simulink model "LATC_Test_Calc"  (R2021b)
settings: Solver=FixedStepDiscrete  StartTime=0.0  StopTime=inf  FixedStep=0.01  RelTol=1e-3
undefined symbols (not defined in the file or in its folder): P_LCS_A0_Dis_BP, P_LCS_A2_Curve_BP, P_LCS_A2S_FliterTime, P_LCS_DeltaEps_SpdBp, P_LCS_LCC_A0_Dis_BP, P_LCS_LCC_AngleSlope_ELK, P_LCS_LCC_AngleSlope_ESS, P_LCS_LCC_AngleSlope_LCCancle, P_LCS_LCC_AngleSlope_LCEco, P_LCS_LCC_AngleSlope_LCK, P_LCS_LCC_AngleSlope_LCKIE, P_LCS_LCC_AngleSlope_LCNomal, P_LCS_LCC_AngleSlope_LCSport, P_LCS_LCC_AngleSlope_LKA, P_LCS_LCC_Eco_AyDtLimit_TBL, P_LCS_LCC_ELK_AyDtLimit_TBL, P_LCS_LCC_ESS_AyDtLimit_TBL, P_LCS_LCC_LC_AyDtLimit_TBL, P_LCS_LCC_LC_Normal_AyDtLimit_TBL, P_LCS_LCC_LC_Planning_Dist_TBL, P_LCS_LCC_LCK_AyDtLimit_TBL, P_LCS_LCC_LCK_Planning_Dist_TBL, P_LCS_LCC_LKA_AyDtLimit_TBL, P_LCS_LCC_Matrix_q1_st, P_LCS_LCC_Matrix_q2_st, P_LCS_LCC_Max_Lateral_Acc_ms2, P_LCS_LCC_MaxLatAcc_ELK, P_LCS_LCC_MaxLatAcc_ESS, P_LCS_LCC_MaxLatAcc_LCCancel, P_LCS_LCC_MaxLatAcc_LCEco, P_LCS_LCC_MaxLatAcc_LCK, P_LCS_LCC_MaxLatAcc_LCKIE, P_LCS_LCC_MaxLatAcc_LCNomal, P_LCS_LCC_MaxLatAcc_LCSport, P_LCS_LCC_MaxLatAcc_LKA, P_LCS_LCC_Min_Plan_Dis, P_LCS_LCC_PlaningLength_m, P_LCS_LCC_PreCur_Min_Plan_Dis_Fac, P_LCS_LCC_PreView_Fac, P_LCS_LCC_PreView_s, P_LCS_LCC_PreViewCurve_Fac, P_LCS_LCC_PreViewT, P_LCS_LCC_Spd_BP, P_LCS_LCC_Spd_BP2, P_LCS_LCC_Sport_AyDtLimit_TBL, P_LCS_LCC_StateActiv_AyDtLimit, P_LCS_LCC_StateActiv_PreviewT, P_LCS_LCC_StateActiveDelaytime, P_LCS_LCC_TarSteerAngleSlope, P_LCS_preDis_spd, P_LCS_StateActiv_AngleSlope, P_LCS_StateActive_HoldTime_BP, P_LCS_StateActiveFlg_BP, P_LCS_StateHold_time
libraries: canapelib x35, simulink x2
(part 2 of 3)

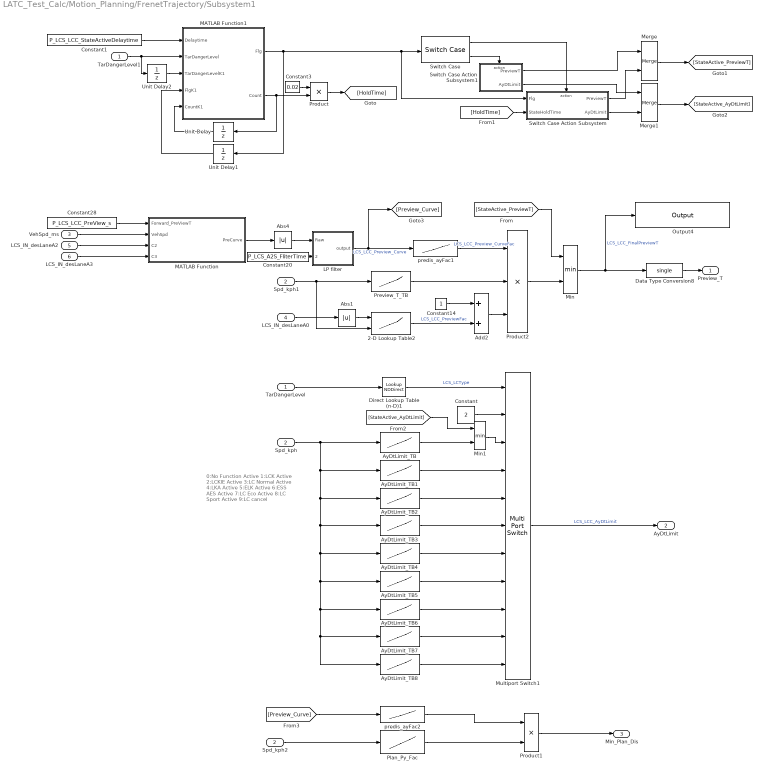
== system LATC_Test_Calc/Motion_Planning/FrenetTrajectory/Subsystem1 ==
  note: 0:No Function Active
      | 1:LCK Active
      | 2:LCKIE Active
      | 3:LC Normal Active
      | 4:LKA Active
      | 5:ELK Active
      | 6:ESS AES Active
      | 7:LC Eco Active
      | 8:LC Sport Active
      | 9:LC cancel
  TarDangerLevel : Inport
  Spd_kph : Inport  Port=2
  VehSpd_ms : Inport  Port=3
  LCS_IN_desLaneA0 : Inport  Port=4
  LCS_IN_desLaneA2 : Inport  Port=5
  LCS_IN_desLaneA3 : Inport  Port=6
  2-D Lookup Table2 : Lookup_n-D  BreakpointsForDimension1=P_LCS_A0_Dis_BP  BreakpointsForDimension2=P_LCS_preDis_spd  Table=P_LCS_LCC_PreView_Fac  ExtrapMethod=Clip  UseLastTableValue=on  InternalRulePriority=Speed  RndMeth=Simplest  InputSameDT=on
      settings: InputPortMap=u0,u1
  Abs1 : Abs
  Abs4 : Abs
  Add2 : Sum
  AyDtLimit_TB : Lookup_n-D  NumberOfTableDimensions=1  BreakpointsForDimension1=P_LCS_preDis_spd  Table=P_LCS_LCC_LCK_AyDtLimit_TBL  ExtrapMethod=Clip  UseLastTableValue=on  InternalRulePriority=Speed  RndMeth=Simplest  InputSameDT=on
  AyDtLimit_TB1 : Lookup_n-D  NumberOfTableDimensions=1  BreakpointsForDimension1=P_LCS_preDis_spd  Table=P_LCS_LCC_LCK_AyDtLimit_TBL  ExtrapMethod=Clip  UseLastTableValue=on  InternalRulePriority=Speed  RndMeth=Simplest  InputSameDT=on
  AyDtLimit_TB2 : Lookup_n-D  NumberOfTableDimensions=1  BreakpointsForDimension1=P_LCS_preDis_spd  Table=P_LCS_LCC_LC_Normal_AyDtLimit_TBL  ExtrapMethod=Clip  UseLastTableValue=on  InternalRulePriority=Speed  RndMeth=Simplest  InputSameDT=on
  AyDtLimit_TB3 : Lookup_n-D  NumberOfTableDimensions=1  BreakpointsForDimension1=P_LCS_preDis_spd  Table=P_LCS_LCC_LKA_AyDtLimit_TBL  ExtrapMethod=Clip  UseLastTableValue=on  InternalRulePriority=Speed  RndMeth=Simplest  InputSameDT=on
  AyDtLimit_TB4 : Lookup_n-D  NumberOfTableDimensions=1  BreakpointsForDimension1=P_LCS_preDis_spd  Table=P_LCS_LCC_ELK_AyDtLimit_TBL  ExtrapMethod=Clip  UseLastTableValue=on  InternalRulePriority=Speed  RndMeth=Simplest  InputSameDT=on
  AyDtLimit_TB5 : Lookup_n-D  NumberOfTableDimensions=1  BreakpointsForDimension1=P_LCS_preDis_spd  Table=P_LCS_LCC_ESS_AyDtLimit_TBL  ExtrapMethod=Clip  UseLastTableValue=on  InternalRulePriority=Speed  RndMeth=Simplest  InputSameDT=on
  AyDtLimit_TB6 : Lookup_n-D  NumberOfTableDimensions=1  BreakpointsForDimension1=P_LCS_preDis_spd  Table=P_LCS_LCC_Eco_AyDtLimit_TBL  ExtrapMethod=Clip  UseLastTableValue=on  InternalRulePriority=Speed  RndMeth=Simplest  InputSameDT=on
  AyDtLimit_TB7 : Lookup_n-D  NumberOfTableDimensions=1  BreakpointsForDimension1=P_LCS_preDis_spd  Table=P_LCS_LCC_Sport_AyDtLimit_TBL  ExtrapMethod=Clip  UseLastTableValue=on  InternalRulePriority=Speed  RndMeth=Simplest  InputSameDT=on
  AyDtLimit_TB8 : Lookup_n-D  NumberOfTableDimensions=1  BreakpointsForDimension1=P_LCS_preDis_spd  Table=P_LCS_LCC_LC_AyDtLimit_TBL  ExtrapMethod=Clip  UseLastTableValue=on  InternalRulePriority=Speed  RndMeth=Simplest  InputSameDT=on
  Constant : Constant  Value=2  OutDataTypeStr=single
  Constant1 : Constant  Value=P_LCS_LCC_StateActiveDelaytime  OutDataTypeStr=uint16
  Constant14 : Constant  OutDataTypeStr=single
  Constant20 : Constant  Value=P_LCS_A2S_FliterTime
  Constant28 : Constant  Value=P_LCS_LCC_PreView_s  OutDataTypeStr=single
  Constant3 : Constant  Value=0.02
  Data Type Conversion8 : DataTypeConversion  OutDataTypeStr=single
  Direct Lookup Table (n-D)1 : LookupNDDirect  NumberOfTableDimensions=1  Table=[0 1 2 3 4 5 6 7 8 9]  TableDataTypeStr=uint8
  LP filter : Subsystem
  MATLAB Function : MATLAB Function  TreatAsAtomicUnit=on
  MATLAB Function1 : MATLAB Function  TreatAsAtomicUnit=on
  Merge : Merge
  Merge1 : Merge
  Min : MinMax  Inputs=2
  Min1 : MinMax  Inputs=2
  Multiport Switch1 : MultiPortSwitch  DataPortOrder=Zero-based contiguous  Inputs=10  zeroidx=on
  Output4 : canapelib/CANape I//O/Output  envName=LCS_LCC_FinalPreviewT  envRows=1  envCols=1  envPortId=0
      settings: AttributesFormatString=%<envName>  SourceProductName=Vector CANape/vSignalyzer Target
  Plan_Py_Fac : Lookup_n-D  NumberOfTableDimensions=1  BreakpointsForDimension1=P_LCS_DeltaEps_SpdBp  Table=P_LCS_LCC_Min_Plan_Dis  ExtrapMethod=Clip  UseLastTableValue=on  InternalRulePriority=Speed  RndMeth=Simplest  InputSameDT=on
  Preview_T_TB : Lookup_n-D  NumberOfTableDimensions=1  BreakpointsForDimension1=P_LCS_preDis_spd  Table=P_LCS_LCC_PreViewT  ExtrapMethod=Clip  UseLastTableValue=on  InternalRulePriority=Speed  RndMeth=Simplest  InputSameDT=on
  Product : Product
  Product1 : Product
  Product2 : Product  Inputs=3
  Spd_kph1 : InportShadow  Port=2
  Spd_kph2 : InportShadow  Port=2
  Switch Case : SwitchCase  CaseConditions={[1]}
  Switch Case Action Subsystem : Subsystem  TreatAsAtomicUnit=on
  Switch Case Action Subsystem1 : Subsystem  TreatAsAtomicUnit=on
  TarDangerLevel1 : InportShadow
  Unit Delay : UnitDelay  SampleTime=-1  HasFrameUpgradeWarning=on
  Unit Delay1 : UnitDelay  SampleTime=-1  HasFrameUpgradeWarning=on
  Unit Delay2 : UnitDelay  SampleTime=-1  HasFrameUpgradeWarning=on
  predis_ayFac1 : Lookup_n-D  NumberOfTableDimensions=1  BreakpointsForDimension1=P_LCS_A2_Curve_BP  Table=P_LCS_LCC_PreViewCurve_Fac  ExtrapMethod=Clip  UseLastTableValue=on  InternalRulePriority=Speed  RndMeth=Simplest  InputSameDT=on
  predis_ayFac2 : Lookup_n-D  NumberOfTableDimensions=1  BreakpointsForDimension1=P_LCS_A2_Curve_BP  Table=P_LCS_LCC_PreCur_Min_Plan_Dis_Fac  ExtrapMethod=Clip  UseLastTableValue=on  InternalRulePriority=Speed  RndMeth=Simplest  InputSameDT=on
  Preview_T : Outport  OutDataTypeStr=single
  AyDtLimit : Outport  Port=2  OutDataTypeStr=single
  Min_Plan_Dis : Outport  Port=3  OutDataTypeStr=single
  wires:
  Min1/1 -> Multiport Switch1/3
  [StateActive_AyDtLimit] -> Min1/1
  Product2/1 -> Min/2
  [StateActive_PreviewT] -> Min/1
  Merge1/1 -> [StateActive_AyDtLimit]
  Merge/1 -> [StateActive_PreviewT]
  Switch Case Action Subsystem1/2(AyDtLimit) -> Merge1/1
  Switch Case Action Subsystem/2(AyDtLimit) -> Merge1/2
  Product/1 -> [HoldTime]
  [HoldTime] -> Switch Case Action Subsystem/2(StateHoldTime)
  Constant3/1 -> Product/1
  Switch Case/2 -> Switch Case Action Subsystem1/Action
  MATLAB Function1/2(Count) -> Unit Delay/1, Product/2
  Switch Case Action Subsystem/1(PreviewT) -> Merge/2
  Switch Case/1 -> Switch Case Action Subsystem/Action
  Switch Case Action Subsystem1/1(PreviewT) -> Merge/1
  MATLAB Function1/1(Flg) -> Switch Case/1, Switch Case Action Subsystem/1(Flg), Unit Delay1/1
  Constant1/1 -> MATLAB Function1/1(Delaytime)
  Unit Delay2/1 -> MATLAB Function1/3(TarDangerLevelK1)
  TarDangerLevel1/1 -> MATLAB Function1/2(TarDangerLevel), Unit Delay2/1
  Unit Delay1/1 -> MATLAB Function1/4(FlgK1)
  Unit Delay/1 -> MATLAB Function1/5(CountK1)
  AyDtLimit_TB8/1 -> Multiport Switch1/11
  AyDtLimit_TB7/1 -> Multiport Switch1/10
  AyDtLimit_TB6/1 -> Multiport Switch1/9
  AyDtLimit_TB5/1 -> Multiport Switch1/8
  AyDtLimit_TB4/1 -> Multiport Switch1/7
  AyDtLimit_TB3/1 -> Multiport Switch1/6
  AyDtLimit_TB2/1 -> Multiport Switch1/5
  AyDtLimit_TB1/1 -> Multiport Switch1/4
  Constant/1 -> Multiport Switch1/2
  Constant28/1 -> MATLAB Function/1(Forward_PreViewT)
  predis_ayFac1/1 -> Product2/1  "LCS_LCC_Preview_CurveFac"
  LP filter/1(output) -> [Preview_Curve], predis_ayFac1/1  "LCS_LCC_Preview_Curve"
  Constant20/1 -> LP filter/2(TorqFilterTime)
  Abs4/1 -> LP filter/1(Raw)
  MATLAB Function/1(PreCurve) -> Abs4/1
  LCS_IN_desLaneA3/1 -> MATLAB Function/4(C3)
  LCS_IN_desLaneA2/1 -> MATLAB Function/3(C2)
  VehSpd_ms/1 -> MATLAB Function/2(VehSpd)
  Data Type Conversion8/1 -> Preview_T/1
  Min/1 -> Output4/1, Data Type Conversion8/1  "LCS_LCC_FinalPreviewT"
  LCS_IN_desLaneA0/1 -> Abs1/1
  Abs1/1 -> 2-D Lookup Table2/1
  Spd_kph1/1 -> Preview_T_TB/1, 2-D Lookup Table2/2
  Add2/1 -> Product2/3
  Constant14/1 -> Add2/1
  2-D Lookup Table2/1 -> Add2/2  "LCS_LCC_PreviewFac"
  Preview_T_TB/1 -> Product2/2
  AyDtLimit_TB/1 -> Min1/2
  Multiport Switch1/1 -> AyDtLimit/1  "LCS_LCC_AyDtLimit"
  Spd_kph/1 -> AyDtLimit_TB/1, AyDtLimit_TB1/1, AyDtLimit_TB2/1, AyDtLimit_TB4/1, AyDtLimit_TB5/1, AyDtLimit_TB7/1, AyDtLimit_TB8/1, AyDtLimit_TB6/1, AyDtLimit_TB3/1
  TarDangerLevel/1 -> Direct Lookup Table (n-D)1/1
  Direct Lookup Table (n-D)1/1 -> Multiport Switch1/1  "LCS_LCType"
  Plan_Py_Fac/1 -> Product1/2
  Spd_kph2/1 -> Plan_Py_Fac/1
  [Preview_Curve] -> predis_ayFac2/1
  Product1/1 -> Min_Plan_Dis/1
  predis_ayFac2/1 -> Product1/1

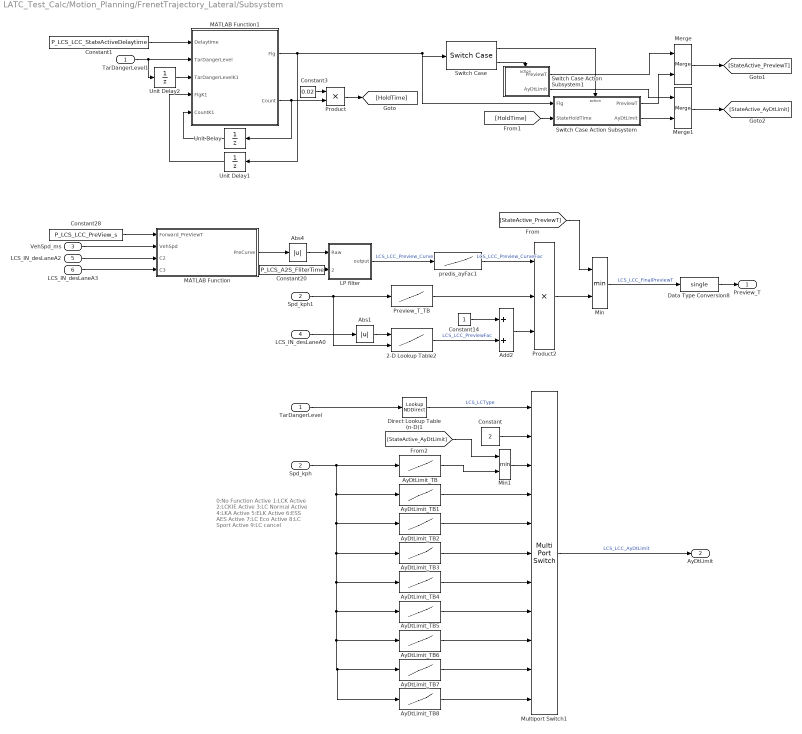
== system LATC_Test_Calc/Motion_Planning/FrenetTrajectory_Lateral/Subsystem ==
  note: 0:No Function Active
      | 1:LCK Active
      | 2:LCKIE Active
      | 3:LC Normal Active
      | 4:LKA Active
      | 5:ELK Active
      | 6:ESS AES Active
      | 7:LC Eco Active
      | 8:LC Sport Active
      | 9:LC cancel
  TarDangerLevel : Inport
  Spd_kph : Inport  Port=2
  VehSpd_ms : Inport  Port=3
  LCS_IN_desLaneA0 : Inport  Port=4
  LCS_IN_desLaneA2 : Inport  Port=5
  LCS_IN_desLaneA3 : Inport  Port=6
  2-D Lookup Table2 : Lookup_n-D  BreakpointsForDimension1=P_LCS_A0_Dis_BP  BreakpointsForDimension2=P_LCS_preDis_spd  Table=P_LCS_LCC_PreView_Fac  ExtrapMethod=Clip  UseLastTableValue=on  InternalRulePriority=Speed  RndMeth=Simplest  InputSameDT=on
      settings: InputPortMap=u0,u1
  Abs1 : Abs
  Abs4 : Abs
  Add2 : Sum
  AyDtLimit_TB : Lookup_n-D  NumberOfTableDimensions=1  BreakpointsForDimension1=P_LCS_preDis_spd  Table=P_LCS_LCC_LCK_AyDtLimit_TBL  ExtrapMethod=Clip  UseLastTableValue=on  InternalRulePriority=Speed  RndMeth=Simplest  InputSameDT=on
  AyDtLimit_TB1 : Lookup_n-D  NumberOfTableDimensions=1  BreakpointsForDimension1=P_LCS_preDis_spd  Table=P_LCS_LCC_LCK_AyDtLimit_TBL  ExtrapMethod=Clip  UseLastTableValue=on  InternalRulePriority=Speed  RndMeth=Simplest  InputSameDT=on
  AyDtLimit_TB2 : Lookup_n-D  NumberOfTableDimensions=1  BreakpointsForDimension1=P_LCS_preDis_spd  Table=P_LCS_LCC_LC_Normal_AyDtLimit_TBL  ExtrapMethod=Clip  UseLastTableValue=on  InternalRulePriority=Speed  RndMeth=Simplest  InputSameDT=on
  AyDtLimit_TB3 : Lookup_n-D  NumberOfTableDimensions=1  BreakpointsForDimension1=P_LCS_preDis_spd  Table=P_LCS_LCC_LKA_AyDtLimit_TBL  ExtrapMethod=Clip  UseLastTableValue=on  InternalRulePriority=Speed  RndMeth=Simplest  InputSameDT=on
  AyDtLimit_TB4 : Lookup_n-D  NumberOfTableDimensions=1  BreakpointsForDimension1=P_LCS_preDis_spd  Table=P_LCS_LCC_ELK_AyDtLimit_TBL  ExtrapMethod=Clip  UseLastTableValue=on  InternalRulePriority=Speed  RndMeth=Simplest  InputSameDT=on
  AyDtLimit_TB5 : Lookup_n-D  NumberOfTableDimensions=1  BreakpointsForDimension1=P_LCS_preDis_spd  Table=P_LCS_LCC_ESS_AyDtLimit_TBL  ExtrapMethod=Clip  UseLastTableValue=on  InternalRulePriority=Speed  RndMeth=Simplest  InputSameDT=on
  AyDtLimit_TB6 : Lookup_n-D  NumberOfTableDimensions=1  BreakpointsForDimension1=P_LCS_preDis_spd  Table=P_LCS_LCC_Eco_AyDtLimit_TBL  ExtrapMethod=Clip  UseLastTableValue=on  InternalRulePriority=Speed  RndMeth=Simplest  InputSameDT=on
  AyDtLimit_TB7 : Lookup_n-D  NumberOfTableDimensions=1  BreakpointsForDimension1=P_LCS_preDis_spd  Table=P_LCS_LCC_Sport_AyDtLimit_TBL  ExtrapMethod=Clip  UseLastTableValue=on  InternalRulePriority=Speed  RndMeth=Simplest  InputSameDT=on
  AyDtLimit_TB8 : Lookup_n-D  NumberOfTableDimensions=1  BreakpointsForDimension1=P_LCS_preDis_spd  Table=P_LCS_LCC_LC_AyDtLimit_TBL  ExtrapMethod=Clip  UseLastTableValue=on  InternalRulePriority=Speed  RndMeth=Simplest  InputSameDT=on
  Constant : Constant  Value=2  OutDataTypeStr=single
  Constant1 : Constant  Value=P_LCS_LCC_StateActiveDelaytime  OutDataTypeStr=uint16
  Constant14 : Constant  OutDataTypeStr=single
  Constant20 : Constant  Value=P_LCS_A2S_FliterTime
  Constant28 : Constant  Value=P_LCS_LCC_PreView_s  OutDataTypeStr=single
  Constant3 : Constant  Value=0.02
  Data Type Conversion8 : DataTypeConversion  OutDataTypeStr=single
  Direct Lookup Table (n-D)1 : LookupNDDirect  NumberOfTableDimensions=1  Table=[0 1 2 3 4 5 6 7 8 9]  TableDataTypeStr=uint8
  LP filter : Subsystem
  MATLAB Function : MATLAB Function  TreatAsAtomicUnit=on
  MATLAB Function1 : MATLAB Function  TreatAsAtomicUnit=on
  Merge : Merge
  Merge1 : Merge
  Min : MinMax  Inputs=2
  Min1 : MinMax  Inputs=2
  Multiport Switch1 : MultiPortSwitch  DataPortOrder=Zero-based contiguous  Inputs=10  zeroidx=on
  Preview_T_TB : Lookup_n-D  NumberOfTableDimensions=1  BreakpointsForDimension1=P_LCS_preDis_spd  Table=P_LCS_LCC_PreViewT  ExtrapMethod=Clip  UseLastTableValue=on  InternalRulePriority=Speed  RndMeth=Simplest  InputSameDT=on
  Product : Product
  Product2 : Product  Inputs=3
  Spd_kph1 : InportShadow  Port=2
  Switch Case : SwitchCase  CaseConditions={[1]}
  Switch Case Action Subsystem : Subsystem  TreatAsAtomicUnit=on
  Switch Case Action Subsystem1 : Subsystem  TreatAsAtomicUnit=on
  TarDangerLevel1 : InportShadow
  Unit Delay : UnitDelay  SampleTime=-1  HasFrameUpgradeWarning=on
  Unit Delay1 : UnitDelay  SampleTime=-1  HasFrameUpgradeWarning=on
  Unit Delay2 : UnitDelay  SampleTime=-1  HasFrameUpgradeWarning=on
  predis_ayFac1 : Lookup_n-D  NumberOfTableDimensions=1  BreakpointsForDimension1=P_LCS_A2_Curve_BP  Table=P_LCS_LCC_PreViewCurve_Fac  ExtrapMethod=Clip  UseLastTableValue=on  InternalRulePriority=Speed  RndMeth=Simplest  InputSameDT=on
  Preview_T : Outport  OutDataTypeStr=single
  AyDtLimit : Outport  Port=2  OutDataTypeStr=single
  wires:
  Direct Lookup Table (n-D)1/1 -> Multiport Switch1/1  "LCS_LCType"
  TarDangerLevel/1 -> Direct Lookup Table (n-D)1/1
  Spd_kph/1 -> AyDtLimit_TB3/1, AyDtLimit_TB6/1, AyDtLimit_TB8/1, AyDtLimit_TB7/1, AyDtLimit_TB5/1, AyDtLimit_TB4/1, AyDtLimit_TB2/1, AyDtLimit_TB1/1, AyDtLimit_TB/1
  Multiport Switch1/1 -> AyDtLimit/1  "LCS_LCC_AyDtLimit"
  AyDtLimit_TB/1 -> Min1/2
  Preview_T_TB/1 -> Product2/2
  2-D Lookup Table2/1 -> Add2/2  "LCS_LCC_PreviewFac"
  Constant14/1 -> Add2/1
  Add2/1 -> Product2/3
  Spd_kph1/1 -> 2-D Lookup Table2/2, Preview_T_TB/1
  Abs1/1 -> 2-D Lookup Table2/1
  LCS_IN_desLaneA0/1 -> Abs1/1
  Min/1 -> Data Type Conversion8/1  "LCS_LCC_FinalPreviewT"
  Data Type Conversion8/1 -> Preview_T/1
  VehSpd_ms/1 -> MATLAB Function/2(VehSpd)
  LCS_IN_desLaneA2/1 -> MATLAB Function/3(C2)
  LCS_IN_desLaneA3/1 -> MATLAB Function/4(C3)
  MATLAB Function/1(PreCurve) -> Abs4/1
  Abs4/1 -> LP filter/1(Raw)
  Constant20/1 -> LP filter/2(TorqFilterTime)
  LP filter/1(output) -> predis_ayFac1/1  "LCS_LCC_Preview_Curve"
  predis_ayFac1/1 -> Product2/1  "LCS_LCC_Preview_CurveFac"
  Constant28/1 -> MATLAB Function/1(Forward_PreViewT)
  Constant/1 -> Multiport Switch1/2
  AyDtLimit_TB1/1 -> Multiport Switch1/4
  AyDtLimit_TB2/1 -> Multiport Switch1/5
  AyDtLimit_TB3/1 -> Multiport Switch1/6
  AyDtLimit_TB4/1 -> Multiport Switch1/7
  AyDtLimit_TB5/1 -> Multiport Switch1/8
  AyDtLimit_TB6/1 -> Multiport Switch1/9
  AyDtLimit_TB7/1 -> Multiport Switch1/10
  AyDtLimit_TB8/1 -> Multiport Switch1/11
  Unit Delay/1 -> MATLAB Function1/5(CountK1)
  Unit Delay1/1 -> MATLAB Function1/4(FlgK1)
  TarDangerLevel1/1 -> Unit Delay2/1, MATLAB Function1/2(TarDangerLevel)
  Unit Delay2/1 -> MATLAB Function1/3(TarDangerLevelK1)
  Constant1/1 -> MATLAB Function1/1(Delaytime)
  MATLAB Function1/1(Flg) -> Unit Delay1/1, Switch Case Action Subsystem/1(Flg), Switch Case/1
  Switch Case Action Subsystem1/1(PreviewT) -> Merge/1
  Switch Case/1 -> Switch Case Action Subsystem/Action
  Switch Case Action Subsystem/1(PreviewT) -> Merge/2
  MATLAB Function1/2(Count) -> Product/2, Unit Delay/1
  Switch Case/2 -> Switch Case Action Subsystem1/Action
  Constant3/1 -> Product/1
  [HoldTime] -> Switch Case Action Subsystem/2(StateHoldTime)
  Product/1 -> [HoldTime]
  Switch Case Action Subsystem/2(AyDtLimit) -> Merge1/2
  Switch Case Action Subsystem1/2(AyDtLimit) -> Merge1/1
  Merge/1 -> [StateActive_PreviewT]
  Merge1/1 -> [StateActive_AyDtLimit]
  [StateActive_PreviewT] -> Min/1
  Product2/1 -> Min/2
  [StateActive_AyDtLimit] -> Min1/1
  Min1/1 -> Multiport Switch1/3

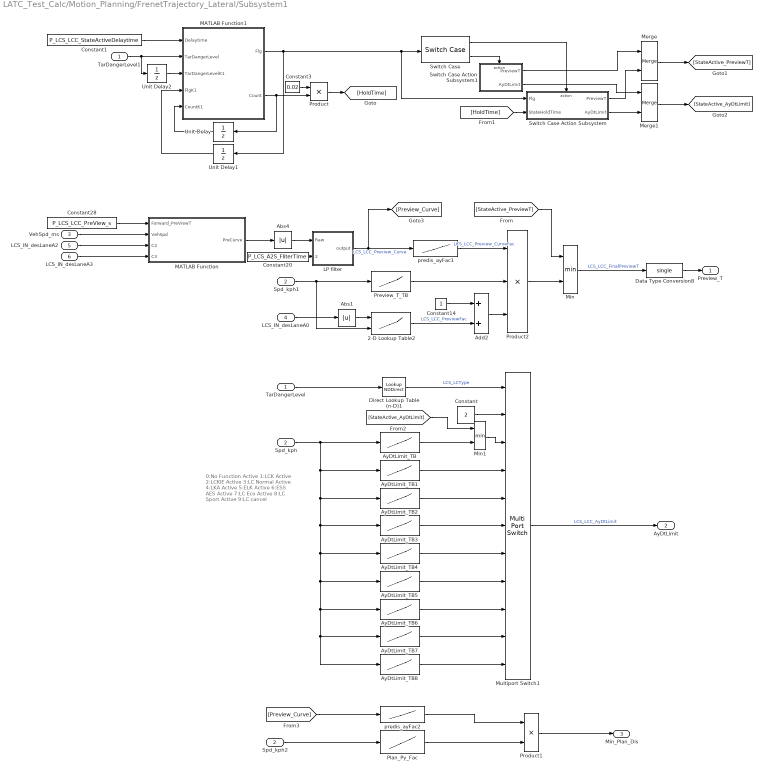
== system LATC_Test_Calc/Motion_Planning/FrenetTrajectory_Lateral/Subsystem1 ==
  note: 0:No Function Active
      | 1:LCK Active
      | 2:LCKIE Active
      | 3:LC Normal Active
      | 4:LKA Active
      | 5:ELK Active
      | 6:ESS AES Active
      | 7:LC Eco Active
      | 8:LC Sport Active
      | 9:LC cancel
  TarDangerLevel : Inport
  Spd_kph : Inport  Port=2
  VehSpd_ms : Inport  Port=3
  LCS_IN_desLaneA0 : Inport  Port=4
  LCS_IN_desLaneA2 : Inport  Port=5
  LCS_IN_desLaneA3 : Inport  Port=6
  2-D Lookup Table2 : Lookup_n-D  BreakpointsForDimension1=P_LCS_A0_Dis_BP  BreakpointsForDimension2=P_LCS_preDis_spd  Table=P_LCS_LCC_PreView_Fac  ExtrapMethod=Clip  UseLastTableValue=on  InternalRulePriority=Speed  RndMeth=Simplest  InputSameDT=on
      settings: InputPortMap=u0,u1
  Abs1 : Abs
  Abs4 : Abs
  Add2 : Sum
  AyDtLimit_TB : Lookup_n-D  NumberOfTableDimensions=1  BreakpointsForDimension1=P_LCS_preDis_spd  Table=P_LCS_LCC_LCK_AyDtLimit_TBL  ExtrapMethod=Clip  UseLastTableValue=on  InternalRulePriority=Speed  RndMeth=Simplest  InputSameDT=on
  AyDtLimit_TB1 : Lookup_n-D  NumberOfTableDimensions=1  BreakpointsForDimension1=P_LCS_preDis_spd  Table=P_LCS_LCC_LCK_AyDtLimit_TBL  ExtrapMethod=Clip  UseLastTableValue=on  InternalRulePriority=Speed  RndMeth=Simplest  InputSameDT=on
  AyDtLimit_TB2 : Lookup_n-D  NumberOfTableDimensions=1  BreakpointsForDimension1=P_LCS_preDis_spd  Table=P_LCS_LCC_LC_Normal_AyDtLimit_TBL  ExtrapMethod=Clip  UseLastTableValue=on  InternalRulePriority=Speed  RndMeth=Simplest  InputSameDT=on
  AyDtLimit_TB3 : Lookup_n-D  NumberOfTableDimensions=1  BreakpointsForDimension1=P_LCS_preDis_spd  Table=P_LCS_LCC_LKA_AyDtLimit_TBL  ExtrapMethod=Clip  UseLastTableValue=on  InternalRulePriority=Speed  RndMeth=Simplest  InputSameDT=on
  AyDtLimit_TB4 : Lookup_n-D  NumberOfTableDimensions=1  BreakpointsForDimension1=P_LCS_preDis_spd  Table=P_LCS_LCC_ELK_AyDtLimit_TBL  ExtrapMethod=Clip  UseLastTableValue=on  InternalRulePriority=Speed  RndMeth=Simplest  InputSameDT=on
  AyDtLimit_TB5 : Lookup_n-D  NumberOfTableDimensions=1  BreakpointsForDimension1=P_LCS_preDis_spd  Table=P_LCS_LCC_ESS_AyDtLimit_TBL  ExtrapMethod=Clip  UseLastTableValue=on  InternalRulePriority=Speed  RndMeth=Simplest  InputSameDT=on
  AyDtLimit_TB6 : Lookup_n-D  NumberOfTableDimensions=1  BreakpointsForDimension1=P_LCS_preDis_spd  Table=P_LCS_LCC_Eco_AyDtLimit_TBL  ExtrapMethod=Clip  UseLastTableValue=on  InternalRulePriority=Speed  RndMeth=Simplest  InputSameDT=on
  AyDtLimit_TB7 : Lookup_n-D  NumberOfTableDimensions=1  BreakpointsForDimension1=P_LCS_preDis_spd  Table=P_LCS_LCC_Sport_AyDtLimit_TBL  ExtrapMethod=Clip  UseLastTableValue=on  InternalRulePriority=Speed  RndMeth=Simplest  InputSameDT=on
  AyDtLimit_TB8 : Lookup_n-D  NumberOfTableDimensions=1  BreakpointsForDimension1=P_LCS_preDis_spd  Table=P_LCS_LCC_LC_AyDtLimit_TBL  ExtrapMethod=Clip  UseLastTableValue=on  InternalRulePriority=Speed  RndMeth=Simplest  InputSameDT=on
  Constant : Constant  Value=2  OutDataTypeStr=single
  Constant1 : Constant  Value=P_LCS_LCC_StateActiveDelaytime  OutDataTypeStr=uint16
  Constant14 : Constant  OutDataTypeStr=single
  Constant20 : Constant  Value=P_LCS_A2S_FliterTime
  Constant28 : Constant  Value=P_LCS_LCC_PreView_s  OutDataTypeStr=single
  Constant3 : Constant  Value=0.02
  Data Type Conversion8 : DataTypeConversion  OutDataTypeStr=single
  Direct Lookup Table (n-D)1 : LookupNDDirect  NumberOfTableDimensions=1  Table=[0 1 2 3 4 5 6 7 8 9]  TableDataTypeStr=uint8
  LP filter : Subsystem
  MATLAB Function : MATLAB Function  TreatAsAtomicUnit=on
  MATLAB Function1 : MATLAB Function  TreatAsAtomicUnit=on
  Merge : Merge
  Merge1 : Merge
  Min : MinMax  Inputs=2
  Min1 : MinMax  Inputs=2
  Multiport Switch1 : MultiPortSwitch  DataPortOrder=Zero-based contiguous  Inputs=10  zeroidx=on
  Plan_Py_Fac : Lookup_n-D  NumberOfTableDimensions=1  BreakpointsForDimension1=P_LCS_DeltaEps_SpdBp  Table=P_LCS_LCC_Min_Plan_Dis  ExtrapMethod=Clip  UseLastTableValue=on  InternalRulePriority=Speed  RndMeth=Simplest  InputSameDT=on
  Preview_T_TB : Lookup_n-D  NumberOfTableDimensions=1  BreakpointsForDimension1=P_LCS_preDis_spd  Table=P_LCS_LCC_PreViewT  ExtrapMethod=Clip  UseLastTableValue=on  InternalRulePriority=Speed  RndMeth=Simplest  InputSameDT=on
  Product : Product
  Product1 : Product
  Product2 : Product  Inputs=3
  Spd_kph1 : InportShadow  Port=2
  Spd_kph2 : InportShadow  Port=2
  Switch Case : SwitchCase  CaseConditions={[1]}
  Switch Case Action Subsystem : Subsystem  TreatAsAtomicUnit=on
  Switch Case Action Subsystem1 : Subsystem  TreatAsAtomicUnit=on
  TarDangerLevel1 : InportShadow
  Unit Delay : UnitDelay  SampleTime=-1  HasFrameUpgradeWarning=on
  Unit Delay1 : UnitDelay  SampleTime=-1  HasFrameUpgradeWarning=on
  Unit Delay2 : UnitDelay  SampleTime=-1  HasFrameUpgradeWarning=on
  predis_ayFac1 : Lookup_n-D  NumberOfTableDimensions=1  BreakpointsForDimension1=P_LCS_A2_Curve_BP  Table=P_LCS_LCC_PreViewCurve_Fac  ExtrapMethod=Clip  UseLastTableValue=on  InternalRulePriority=Speed  RndMeth=Simplest  InputSameDT=on
  predis_ayFac2 : Lookup_n-D  NumberOfTableDimensions=1  BreakpointsForDimension1=P_LCS_A2_Curve_BP  Table=P_LCS_LCC_PreCur_Min_Plan_Dis_Fac  ExtrapMethod=Clip  UseLastTableValue=on  InternalRulePriority=Speed  RndMeth=Simplest  InputSameDT=on
  Preview_T : Outport  OutDataTypeStr=single
  AyDtLimit : Outport  Port=2  OutDataTypeStr=single
  Min_Plan_Dis : Outport  Port=3  OutDataTypeStr=single
  wires:
  Min1/1 -> Multiport Switch1/3
  [StateActive_AyDtLimit] -> Min1/1
  Product2/1 -> Min/2
  [StateActive_PreviewT] -> Min/1
  Merge1/1 -> [StateActive_AyDtLimit]
  Merge/1 -> [StateActive_PreviewT]
  Switch Case Action Subsystem1/2(AyDtLimit) -> Merge1/1
  Switch Case Action Subsystem/2(AyDtLimit) -> Merge1/2
  Product/1 -> [HoldTime]
  [HoldTime] -> Switch Case Action Subsystem/2(StateHoldTime)
  Constant3/1 -> Product/1
  Switch Case/2 -> Switch Case Action Subsystem1/Action
  MATLAB Function1/2(Count) -> Unit Delay/1, Product/2
  Switch Case Action Subsystem/1(PreviewT) -> Merge/2
  Switch Case/1 -> Switch Case Action Subsystem/Action
  Switch Case Action Subsystem1/1(PreviewT) -> Merge/1
  MATLAB Function1/1(Flg) -> Switch Case/1, Switch Case Action Subsystem/1(Flg), Unit Delay1/1
  Constant1/1 -> MATLAB Function1/1(Delaytime)
  Unit Delay2/1 -> MATLAB Function1/3(TarDangerLevelK1)
  TarDangerLevel1/1 -> MATLAB Function1/2(TarDangerLevel), Unit Delay2/1
  Unit Delay1/1 -> MATLAB Function1/4(FlgK1)
  Unit Delay/1 -> MATLAB Function1/5(CountK1)
  AyDtLimit_TB8/1 -> Multiport Switch1/11
  AyDtLimit_TB7/1 -> Multiport Switch1/10
  AyDtLimit_TB6/1 -> Multiport Switch1/9
  AyDtLimit_TB5/1 -> Multiport Switch1/8
  AyDtLimit_TB4/1 -> Multiport Switch1/7
  AyDtLimit_TB3/1 -> Multiport Switch1/6
  AyDtLimit_TB2/1 -> Multiport Switch1/5
  AyDtLimit_TB1/1 -> Multiport Switch1/4
  Constant/1 -> Multiport Switch1/2
  Constant28/1 -> MATLAB Function/1(Forward_PreViewT)
  predis_ayFac1/1 -> Product2/1  "LCS_LCC_Preview_CurveFac"
  LP filter/1(output) -> [Preview_Curve], predis_ayFac1/1  "LCS_LCC_Preview_Curve"
  Constant20/1 -> LP filter/2(TorqFilterTime)
  Abs4/1 -> LP filter/1(Raw)
  MATLAB Function/1(PreCurve) -> Abs4/1
  LCS_IN_desLaneA3/1 -> MATLAB Function/4(C3)
  LCS_IN_desLaneA2/1 -> MATLAB Function/3(C2)
  VehSpd_ms/1 -> MATLAB Function/2(VehSpd)
  Data Type Conversion8/1 -> Preview_T/1
  Min/1 -> Data Type Conversion8/1  "LCS_LCC_FinalPreviewT"
  LCS_IN_desLaneA0/1 -> Abs1/1
  Abs1/1 -> 2-D Lookup Table2/1
  Spd_kph1/1 -> Preview_T_TB/1, 2-D Lookup Table2/2
  Add2/1 -> Product2/3
  Constant14/1 -> Add2/1
  2-D Lookup Table2/1 -> Add2/2  "LCS_LCC_PreviewFac"
  Preview_T_TB/1 -> Product2/2
  AyDtLimit_TB/1 -> Min1/2
  Multiport Switch1/1 -> AyDtLimit/1  "LCS_LCC_AyDtLimit"
  Spd_kph/1 -> AyDtLimit_TB/1, AyDtLimit_TB1/1, AyDtLimit_TB2/1, AyDtLimit_TB4/1, AyDtLimit_TB5/1, AyDtLimit_TB7/1, AyDtLimit_TB8/1, AyDtLimit_TB6/1, AyDtLimit_TB3/1
  TarDangerLevel/1 -> Direct Lookup Table (n-D)1/1
  Direct Lookup Table (n-D)1/1 -> Multiport Switch1/1  "LCS_LCType"
  Plan_Py_Fac/1 -> Product1/2
  Spd_kph2/1 -> Plan_Py_Fac/1
  [Preview_Curve] -> predis_ayFac2/1
  Product1/1 -> Min_Plan_Dis/1
  predis_ayFac2/1 -> Product1/1

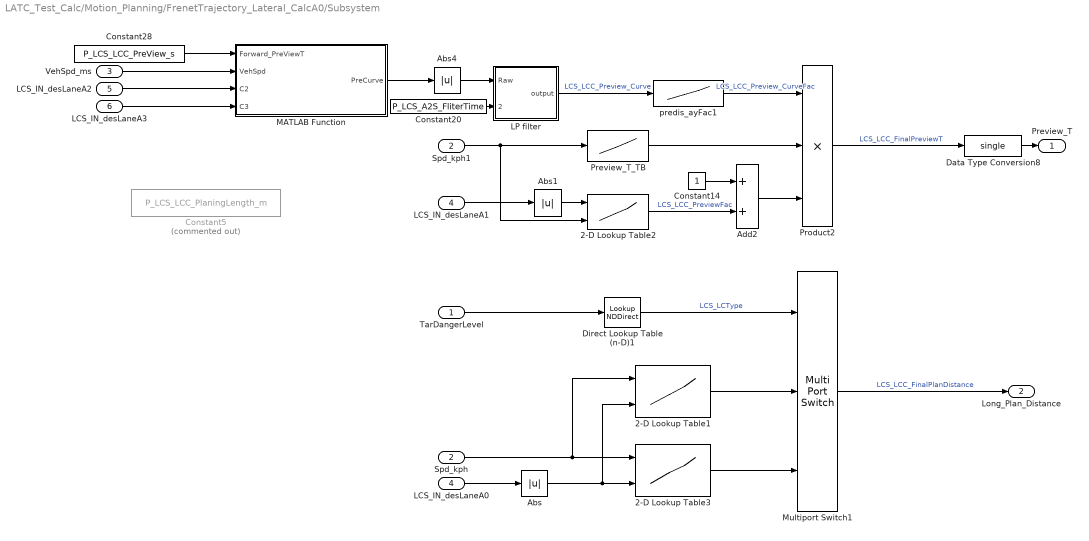
== system LATC_Test_Calc/Motion_Planning/FrenetTrajectory_Lateral_CalcA0/Subsystem ==
  TarDangerLevel : Inport
  Spd_kph : Inport  Port=2
  VehSpd_ms : Inport  Port=3
  LCS_IN_desLaneA0 : Inport  Port=4
  LCS_IN_desLaneA2 : Inport  Port=5
  LCS_IN_desLaneA3 : Inport  Port=6
  2-D Lookup Table1 : Lookup_n-D  BreakpointsForDimension1=P_LCS_LCC_Spd_BP2  BreakpointsForDimension2=P_LCS_LCC_A0_Dis_BP  Table=P_LCS_LCC_LCK_Planning_Dist_TBL  ExtrapMethod=Clip  UseLastTableValue=on  InternalRulePriority=Speed  RndMeth=Simplest  InputSameDT=on
      settings: InputPortMap=u0,u1
  2-D Lookup Table2 : Lookup_n-D  BreakpointsForDimension1=P_LCS_A0_Dis_BP  BreakpointsForDimension2=P_LCS_preDis_spd  Table=P_LCS_LCC_PreView_Fac  ExtrapMethod=Clip  UseLastTableValue=on  InternalRulePriority=Speed  RndMeth=Simplest  InputSameDT=on
      settings: InputPortMap=u0,u1
  2-D Lookup Table3 : Lookup_n-D  BreakpointsForDimension1=P_LCS_LCC_Spd_BP  BreakpointsForDimension2=P_LCS_LCC_A0_Dis_BP  Table=P_LCS_LCC_LC_Planning_Dist_TBL  ExtrapMethod=Clip  UseLastTableValue=on  InternalRulePriority=Speed  RndMeth=Simplest  InputSameDT=on
      settings: InputPortMap=u0,u1
  Abs : Abs
  Abs1 : Abs
  Abs4 : Abs
  Add2 : Sum
  Constant14 : Constant  OutDataTypeStr=single
  Constant20 : Constant  Value=P_LCS_A2S_FliterTime
  Constant28 : Constant  Value=P_LCS_LCC_PreView_s  OutDataTypeStr=single
  Constant5 : Constant  Commented=on  Value=P_LCS_LCC_PlaningLength_m  OutDataTypeStr=single
  Data Type Conversion8 : DataTypeConversion  OutDataTypeStr=single
  Direct Lookup Table (n-D)1 : LookupNDDirect  NumberOfTableDimensions=1  Table=[1 1 1 2 1 1 1 2 2 1 1]  TableDataTypeStr=uint8
  LCS_IN_desLaneA1 : InportShadow  Port=4
  LP filter : Subsystem
  MATLAB Function : MATLAB Function  TreatAsAtomicUnit=on
  Multiport Switch1 : MultiPortSwitch  Inputs=2
  Preview_T_TB : Lookup_n-D  NumberOfTableDimensions=1  BreakpointsForDimension1=P_LCS_preDis_spd  Table=P_LCS_LCC_PreViewT  ExtrapMethod=Clip  UseLastTableValue=on  InternalRulePriority=Speed  RndMeth=Simplest  InputSameDT=on
  Product2 : Product  Inputs=3
  Spd_kph1 : InportShadow  Port=2
  predis_ayFac1 : Lookup_n-D  NumberOfTableDimensions=1  BreakpointsForDimension1=P_LCS_A2_Curve_BP  Table=P_LCS_LCC_PreViewCurve_Fac  ExtrapMethod=Clip  UseLastTableValue=on  InternalRulePriority=Speed  RndMeth=Simplest  InputSameDT=on
  Preview_T : Outport  OutDataTypeStr=single
  Long_Plan_Distance : Outport  Port=2  OutDataTypeStr=single
  wires:
  2-D Lookup Table1/1 -> Multiport Switch1/2
  Direct Lookup Table (n-D)1/1 -> Multiport Switch1/1  "LCS_LCType"
  TarDangerLevel/1 -> Direct Lookup Table (n-D)1/1
  Spd_kph/1 -> 2-D Lookup Table1/1, 2-D Lookup Table3/1
  LCS_IN_desLaneA0/1 -> Abs/1
  Abs/1 -> 2-D Lookup Table1/2, 2-D Lookup Table3/2
  Multiport Switch1/1 -> Long_Plan_Distance/1  "LCS_LCC_FinalPlanDistance"
  2-D Lookup Table3/1 -> Multiport Switch1/3
  Preview_T_TB/1 -> Product2/2
  2-D Lookup Table2/1 -> Add2/2  "LCS_LCC_PreviewFac"
  Constant14/1 -> Add2/1
  Add2/1 -> Product2/3
  Spd_kph1/1 -> 2-D Lookup Table2/2, Preview_T_TB/1
  Abs1/1 -> 2-D Lookup Table2/1
  LCS_IN_desLaneA1/1 -> Abs1/1
  Product2/1 -> Data Type Conversion8/1  "LCS_LCC_FinalPreviewT"
  Data Type Conversion8/1 -> Preview_T/1
  VehSpd_ms/1 -> MATLAB Function/2(VehSpd)
  LCS_IN_desLaneA2/1 -> MATLAB Function/3(C2)
  LCS_IN_desLaneA3/1 -> MATLAB Function/4(C3)
  MATLAB Function/1(PreCurve) -> Abs4/1
  Abs4/1 -> LP filter/1(Raw)
  Constant20/1 -> LP filter/2(TorqFilterTime)
  LP filter/1(output) -> predis_ayFac1/1  "LCS_LCC_Preview_Curve"
  predis_ayFac1/1 -> Product2/1  "LCS_LCC_Preview_CurveFac"
  Constant28/1 -> MATLAB Function/1(Forward_PreViewT)

== system LATC_Test_Calc/Motion_Planning/CartesianTrajectory/Subsystem/LP filter ==
  Raw : Inport
  TorqFilterTime : Inport  Port=2
  Memory2 : Memory  InheritSampleTime=on
  Product1 : Product  RndMeth=Zero
  Product4 : Product  Inputs=*/  RndMeth=Zero
  Sum4 : Sum  Inputs=+-|
  Sum5 : Sum  Inputs=++|
  Weight/N3 : Constant  Value=0.02  OutDataTypeStr=single
  output : Outport
  wires:
  TorqFilterTime/1 -> Product4/2
  Product4/1 -> Product1/1
  Weight/N3/1 -> Product4/1
  Raw/1 -> Sum4/1
  Product1/1 -> Sum5/1
  Sum4/1 -> Product1/2
  Memory2/1 -> Sum4/2, Sum5/2
  Sum5/1 -> output/1, Memory2/1

== system LATC_Test_Calc/Motion_Planning/CartesianTrajectory/Subsystem/Switch Case Action Subsystem ==
  Flg : Inport
  StateHoldTime : Inport  Port=2
  Action Port : ActionPort  ActionPortLabel=case [ 1 ]:
  ActiveAyDtLimit_TBL : Lookup_n-D  BreakpointsForDimension1=P_LCS_StateActiveFlg_BP  BreakpointsForDimension2=P_LCS_StateActive_HoldTime_BP  Table=P_LCS_LCC_StateActiv_AyDtLimit  ExtrapMethod=Clip  UseLastTableValue=on  InternalRulePriority=Speed  OutDataTypeStr=single  RndMeth=Simplest
      settings: InputPortMap=u0,u1
  ActivePreviewT_TBL : Lookup_n-D  BreakpointsForDimension1=P_LCS_StateActiveFlg_BP  BreakpointsForDimension2=P_LCS_StateActive_HoldTime_BP  Table=P_LCS_LCC_StateActiv_PreviewT  ExtrapMethod=Clip  UseLastTableValue=on  InternalRulePriority=Speed  OutDataTypeStr=single  RndMeth=Simplest
      settings: InputPortMap=u0,u1
  PreviewT : Outport
  AyDtLimit : Outport  Port=2
  wires:
  ActiveAyDtLimit_TBL/1 -> AyDtLimit/1
  Flg/1 -> ActivePreviewT_TBL/1, ActiveAyDtLimit_TBL/1
  ActivePreviewT_TBL/1 -> PreviewT/1
  StateHoldTime/1 -> ActivePreviewT_TBL/2, ActiveAyDtLimit_TBL/2

== system LATC_Test_Calc/Motion_Planning/CartesianTrajectory/Subsystem/Switch Case Action Subsystem1 ==
  Action Port : ActionPort  ActionPortLabel=default:
  Constant : Constant  Value=10  OutDataTypeStr=single
  Constant1 : Constant  Value=10  OutDataTypeStr=single
  PreviewT : Outport
  AyDtLimit : Outport  Port=2
  wires:
  Constant1/1 -> AyDtLimit/1
  Constant/1 -> PreviewT/1

== system LATC_Test_Calc/Motion_Planning/FrenetTrajectory/Subsystem1/LP filter ==
  Raw : Inport
  TorqFilterTime : Inport  Port=2
  Memory2 : Memory  InheritSampleTime=on
  Product1 : Product  RndMeth=Zero
  Product4 : Product  Inputs=*/  RndMeth=Zero
  Sum4 : Sum  Inputs=+-|
  Sum5 : Sum  Inputs=++|
  Weight/N3 : Constant  Value=0.02  OutDataTypeStr=single
  output : Outport
  wires:
  TorqFilterTime/1 -> Product4/2
  Product4/1 -> Product1/1
  Weight/N3/1 -> Product4/1
  Raw/1 -> Sum4/1
  Product1/1 -> Sum5/1
  Sum4/1 -> Product1/2
  Memory2/1 -> Sum4/2, Sum5/2
  Sum5/1 -> output/1, Memory2/1

== system LATC_Test_Calc/Motion_Planning/FrenetTrajectory/Subsystem1/Switch Case Action Subsystem ==
  Flg : Inport
  StateHoldTime : Inport  Port=2
  Action Port : ActionPort  ActionPortLabel=case [ 1 ]:
  ActiveAyDtLimit_TBL : Lookup_n-D  BreakpointsForDimension1=P_LCS_StateActiveFlg_BP  BreakpointsForDimension2=P_LCS_StateActive_HoldTime_BP  Table=P_LCS_LCC_StateActiv_AyDtLimit  ExtrapMethod=Clip  UseLastTableValue=on  InternalRulePriority=Speed  OutDataTypeStr=single  RndMeth=Simplest
      settings: InputPortMap=u0,u1
  ActivePreviewT_TBL : Lookup_n-D  BreakpointsForDimension1=P_LCS_StateActiveFlg_BP  BreakpointsForDimension2=P_LCS_StateActive_HoldTime_BP  Table=P_LCS_LCC_StateActiv_PreviewT  ExtrapMethod=Clip  UseLastTableValue=on  InternalRulePriority=Speed  OutDataTypeStr=single  RndMeth=Simplest
      settings: InputPortMap=u0,u1
  PreviewT : Outport
  AyDtLimit : Outport  Port=2
  wires:
  ActiveAyDtLimit_TBL/1 -> AyDtLimit/1
  Flg/1 -> ActivePreviewT_TBL/1, ActiveAyDtLimit_TBL/1
  ActivePreviewT_TBL/1 -> PreviewT/1
  StateHoldTime/1 -> ActivePreviewT_TBL/2, ActiveAyDtLimit_TBL/2

== system LATC_Test_Calc/Motion_Planning/FrenetTrajectory/Subsystem1/Switch Case Action Subsystem1 ==
  Action Port : ActionPort  ActionPortLabel=default:
  Constant : Constant  Value=10  OutDataTypeStr=single
  Constant1 : Constant  Value=10  OutDataTypeStr=single
  PreviewT : Outport
  AyDtLimit : Outport  Port=2
  wires:
  Constant1/1 -> AyDtLimit/1
  Constant/1 -> PreviewT/1

== system LATC_Test_Calc/Motion_Planning/FrenetTrajectory_Lateral/Subsystem/LP filter ==
  Raw : Inport
  TorqFilterTime : Inport  Port=2
  Memory2 : Memory  InheritSampleTime=on
  Product1 : Product  RndMeth=Zero
  Product4 : Product  Inputs=*/  RndMeth=Zero
  Sum4 : Sum  Inputs=+-|
  Sum5 : Sum  Inputs=++|
  Weight/N3 : Constant  Value=0.02  OutDataTypeStr=single
  output : Outport
  wires:
  Sum5/1 -> Memory2/1, output/1
  Memory2/1 -> Sum5/2, Sum4/2
  Sum4/1 -> Product1/2
  Product1/1 -> Sum5/1
  Raw/1 -> Sum4/1
  Weight/N3/1 -> Product4/1
  Product4/1 -> Product1/1
  TorqFilterTime/1 -> Product4/2

== system LATC_Test_Calc/Motion_Planning/FrenetTrajectory_Lateral/Subsystem/Switch Case Action Subsystem ==
  Flg : Inport
  StateHoldTime : Inport  Port=2
  Action Port : ActionPort
  ActiveAyDtLimit_TBL : Lookup_n-D  BreakpointsForDimension1=P_LCS_StateActiveFlg_BP  BreakpointsForDimension2=P_LCS_StateActive_HoldTime_BP  Table=P_LCS_LCC_StateActiv_AyDtLimit  ExtrapMethod=Clip  UseLastTableValue=on  InternalRulePriority=Speed  OutDataTypeStr=single  RndMeth=Simplest
      settings: InputPortMap=u0,u1
  ActivePreviewT_TBL : Lookup_n-D  BreakpointsForDimension1=P_LCS_StateActiveFlg_BP  BreakpointsForDimension2=P_LCS_StateActive_HoldTime_BP  Table=P_LCS_LCC_StateActiv_PreviewT  ExtrapMethod=Clip  UseLastTableValue=on  InternalRulePriority=Speed  OutDataTypeStr=single  RndMeth=Simplest
      settings: InputPortMap=u0,u1
  PreviewT : Outport
  AyDtLimit : Outport  Port=2
  wires:
  StateHoldTime/1 -> ActiveAyDtLimit_TBL/2, ActivePreviewT_TBL/2
  ActivePreviewT_TBL/1 -> PreviewT/1
  Flg/1 -> ActiveAyDtLimit_TBL/1, ActivePreviewT_TBL/1
  ActiveAyDtLimit_TBL/1 -> AyDtLimit/1

== system LATC_Test_Calc/Motion_Planning/FrenetTrajectory_Lateral/Subsystem/Switch Case Action Subsystem1 ==
  Action Port : ActionPort
  Constant : Constant  Value=10  OutDataTypeStr=single
  Constant1 : Constant  Value=10  OutDataTypeStr=single
  PreviewT : Outport
  AyDtLimit : Outport  Port=2
  wires:
  Constant/1 -> PreviewT/1
  Constant1/1 -> AyDtLimit/1

== system LATC_Test_Calc/Motion_Planning/FrenetTrajectory_Lateral/Subsystem1/LP filter ==
  Raw : Inport
  TorqFilterTime : Inport  Port=2
  Memory2 : Memory  InheritSampleTime=on
  Product1 : Product  RndMeth=Zero
  Product4 : Product  Inputs=*/  RndMeth=Zero
  Sum4 : Sum  Inputs=+-|
  Sum5 : Sum  Inputs=++|
  Weight/N3 : Constant  Value=0.02  OutDataTypeStr=single
  output : Outport
  wires:
  TorqFilterTime/1 -> Product4/2
  Product4/1 -> Product1/1
  Weight/N3/1 -> Product4/1
  Raw/1 -> Sum4/1
  Product1/1 -> Sum5/1
  Sum4/1 -> Product1/2
  Memory2/1 -> Sum4/2, Sum5/2
  Sum5/1 -> output/1, Memory2/1

== system LATC_Test_Calc/Motion_Planning/FrenetTrajectory_Lateral/Subsystem1/Switch Case Action Subsystem ==
  Flg : Inport
  StateHoldTime : Inport  Port=2
  Action Port : ActionPort  ActionPortLabel=case [ 1 ]:
  ActiveAyDtLimit_TBL : Lookup_n-D  BreakpointsForDimension1=P_LCS_StateActiveFlg_BP  BreakpointsForDimension2=P_LCS_StateActive_HoldTime_BP  Table=P_LCS_LCC_StateActiv_AyDtLimit  ExtrapMethod=Clip  UseLastTableValue=on  InternalRulePriority=Speed  OutDataTypeStr=single  RndMeth=Simplest
      settings: InputPortMap=u0,u1
  ActivePreviewT_TBL : Lookup_n-D  BreakpointsForDimension1=P_LCS_StateActiveFlg_BP  BreakpointsForDimension2=P_LCS_StateActive_HoldTime_BP  Table=P_LCS_LCC_StateActiv_PreviewT  ExtrapMethod=Clip  UseLastTableValue=on  InternalRulePriority=Speed  OutDataTypeStr=single  RndMeth=Simplest
      settings: InputPortMap=u0,u1
  PreviewT : Outport
  AyDtLimit : Outport  Port=2
  wires:
  ActiveAyDtLimit_TBL/1 -> AyDtLimit/1
  Flg/1 -> ActivePreviewT_TBL/1, ActiveAyDtLimit_TBL/1
  ActivePreviewT_TBL/1 -> PreviewT/1
  StateHoldTime/1 -> ActivePreviewT_TBL/2, ActiveAyDtLimit_TBL/2

== system LATC_Test_Calc/Motion_Planning/FrenetTrajectory_Lateral/Subsystem1/Switch Case Action Subsystem1 ==
  Action Port : ActionPort  ActionPortLabel=default:
  Constant : Constant  Value=10  OutDataTypeStr=single
  Constant1 : Constant  Value=10  OutDataTypeStr=single
  PreviewT : Outport
  AyDtLimit : Outport  Port=2
  wires:
  Constant1/1 -> AyDtLimit/1
  Constant/1 -> PreviewT/1

== system LATC_Test_Calc/Motion_Planning/FrenetTrajectory_Lateral_CalcA0/Subsystem/LP filter ==
  Raw : Inport
  TorqFilterTime : Inport  Port=2
  Memory2 : Memory  InheritSampleTime=on
  Product1 : Product  RndMeth=Zero
  Product4 : Product  Inputs=*/  RndMeth=Zero
  Sum4 : Sum  Inputs=+-|
  Sum5 : Sum  Inputs=++|
  Weight/N3 : Constant  Value=0.02  OutDataTypeStr=single
  output : Outport
  wires:
  Sum5/1 -> Memory2/1, output/1
  Memory2/1 -> Sum5/2, Sum4/2
  Sum4/1 -> Product1/2
  Product1/1 -> Sum5/1
  Raw/1 -> Sum4/1
  Weight/N3/1 -> Product4/1
  Product4/1 -> Product1/1
  TorqFilterTime/1 -> Product4/2

== matlab function LATC_Test_Calc/Motion_Planning/FrenetTrajectory/Subsystem1/MATLAB Function ==
  data: Forward_PreViewT input; VehSpd input; PreCurve output; C2 input; C3 input
function PreCurve = PreView_Point_Curvature(Forward_PreViewT,VehSpd,C2,C3)
LookForwardDis = VehSpd * Forward_PreViewT;
PreCurve = 6*C3*LookForwardDis + 2*C2;
end

== matlab function LATC_Test_Calc/Motion_Planning/FrenetTrajectory_Lateral_CalcA0/MATLAB Function4 ==
  data: A0 input; A1 input; A2 input; A3 input; Veh_Speed input size=1; YawRate input size=1; PreView_T input size=1; PlanX output; PlanY output; PlanTheta output; idx output; PreviewX output; PreviewY output; PreviewTheta output; numTraj output size=1; ref_curvature output; arcLenOffsets input size=1; lateral_error output size=1; lateral_error_rate output size=1; heading_error output size=1; heading_error_rate output size=1; TarDangerlLevel input
function [PlanX,PlanY,PlanTheta,idx,PreviewX,PreviewY,PreviewTheta,numTraj,ref_curvature,lateral_error,lateral_error_rate,heading_error,heading_error_rate]= fcn(A0,A1,A2,A3,Veh_Speed,YawRate,PreView_T,arcLenOffsets,TarDangerlLevel)
% 参考线离散化
rx1 = [single(0):single(1):single(9)];
rx2 = [single(10):20:150];
rx = cat(2,rx1,rx2);
ry = single((-1)).*(A0 + A1.* rx + A2.* (rx.^2) + A3.* (rx.^3));
waypoints = [ry',rx'];
referencePath = FrenentReferencePath(waypoints,20);
pathStart = referencePath.interpolate(0);% 求起始点处车辆状态 [x, y,theta, kappa, dkappa, s]
initialState=[0 -A0 pathStart(1,3)];

Frenet_traj_obj = TrajectoryGeneratorFrenet(referencePath);
FtNumTarpoints = single(40); % Frenet坐标系轨迹点数
GtNumTarpoints = single(40); % 全局坐标系轨迹点数
%% 生成轨迹
if abs(A0)<single(0.2) && (TarDangerlLevel ~= 3 ||TarDangerlLevel ~= 6 || TarDangerlLevel ~= 7 || TarDangerlLevel ~= 8 )
    globaltraj = single(zeros(40,5));
    costs = single(zeros(1,1));
    globalTrajectory = struct('Trajectory',globaltraj,'costs',costs);
    rx_Traj = [single(0):single(2):single(80)];
    ry_Traj = single((-1)).*(A0 + A1.* rx_Traj + A2.* (rx_Traj.^2) + A3.* (rx_Traj.^3));
    Traj_objSpline = Spline2D(ry_Traj,rx_Traj);
    s_Traj = linspace(single(0),single(60),40);
    TargetPoints = single(zeros(length(s_Traj),5));
    for i = single(1):single(1):length(s_Traj)
        [ix,iy] = Traj_objSpline.calc_position(s_Traj(i));
        TargetPoints(i,1) = ix;
        TargetPoints(i,2) = iy;
        TargetPoints(i,3) = Traj_objSpline.calc_yaw(s_Traj(i));
        TargetPoints(i,4) = Traj_objSpline.calc_curvature(s_Traj(i));
        TargetPoints(i,5) = Traj_objSpline.calc_curvatureDerivative(s_Traj(i));
    end
    globalTrajectory.Trajectory = TargetPoints;
    numTraj  = 0;
else
    [frenetTrajectory,globalTrajectory,numTraj] = Frenet_traj_obj.FrenetTrajectory_Lateral(initialState,arcLenOffsets,0,FtNumTarpoints,GtNumTarpoints);
    [globalTrajectory] = EvaluateTrajectory_Lateral(frenetTrajectory,globalTrajectory, 1,1);
end
%%
% [s,d]→[x, y, theta, kappa, dkappa]
PlanX = single(zeros(40,1));
PlanY = single(zeros(40,1));
PlanTheta = single(zeros(40,1));
PlanX= globalTrajectory(1).Trajectory(1:40,2);
PlanY= globalTrajectory(1).Trajectory(1:40,1);
PlanTheta = globalTrajectory(1).Trajectory(1:40,3);
[matrix_state,ref_curvature,idx] = Calc_State_Error(Veh_Speed,YawRate,globalTrajectory,PreView_T);
PreviewX = globalTrajectory(1).Trajectory(idx,2);
PreviewY = globalTrajectory(1).Trajectory(idx,1);
PreviewTheta = globalTrajectory(1).Trajectory(idx,3);
% lateral_error = single(zeros(1,1));lateral_error_rate = single(zeros(1,1));heading_error = single(zeros(1,1));heading_error_rate = single(zeros(1,1));
lateral_error = matrix_state(1,1);
lateral_error_rate = matrix_state(2,1);
heading_error = matrix_state(3,1);
heading_error_rate = matrix_state(4,1);

end

== matlab function LATC_Test_Calc/Motion_Planning/FrenetTrajectory/Subsystem1/MATLAB Function1 ==
  data: Delaytime input uint16; Flg output uint8; Count output uint16; TarDangerLevel input uint8; TarDangerLevelK1 input uint8; FlgK1 input uint8; CountK1 input uint16
function [Flg,Count]= fcn(Delaytime,TarDangerLevel,TarDangerLevelK1,FlgK1,CountK1)
Count = min(CountK1 + uint16(1),Delaytime);
if Count == Delaytime
    Flg = uint8(0);
else
    Flg = FlgK1;
end
%%状态检测
if TarDangerLevel == uint8(1) && TarDangerLevelK1 == 0 %功能激活
    Count = uint16(0);
    Flg = uint8(1);  
end
end
